simulink model "Manager_1"  (R2025b)
settings: configuration reference "code" (kept outside this file)
undefined symbols (not defined in the file or in its folder): Button, buttonValue, TsControl
settings Model: DataDictionary=test.sldd  Creator=rpumpo  LastModifiedBy=rpumpo
settings ConfigSetRef: SourceName=code

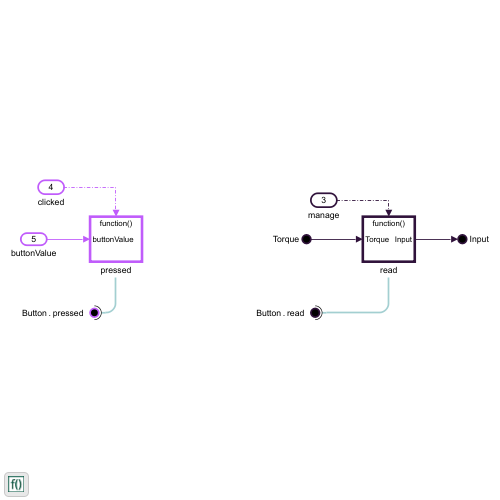
[thumbnail: Simulink's stored preview of the top-level diagram]
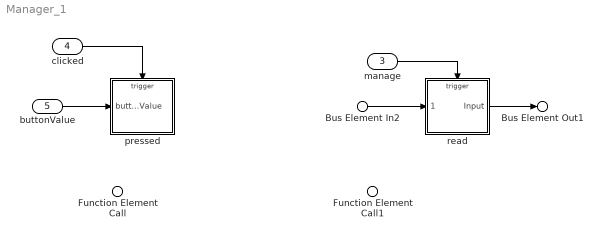
== system Manager_1 ==
  Function Element Call1 : Inport  AllowServiceAccess=on  PortName=Button  Element=read
  Function Element Call : Inport  AllowServiceAccess=on  PortName=Button  Element=pressed
  Bus Element In2 : Inport  Port=2  PortName=Torque
  manage : Inport  Port=3  SampleTime=TsControl  OutputFunctionCall=on
  clicked : Inport  Port=4  OutputFunctionCall=on
  buttonValue : Inport  Port=5
  pressed : Subsystem
  read : Subsystem
  Bus Element Out1 : Outport  PortName=Input
  wires:
  manage/1 -> read/Trigger
  read/1(Input) -> Bus Element Out1/1
  Bus Element In2/1 -> read/1(Torque)
  clicked/1 -> pressed/Trigger
  buttonValue/1 -> pressed/1(buttonValue)

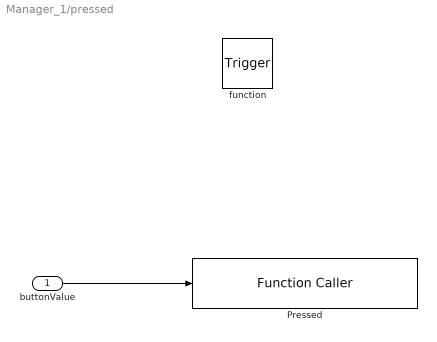
== system Manager_1/pressed ==
  buttonValue : Inport
  function : TriggerPort  TriggerType=function-call  VariantControl=(inherit)
  Pressed : FunctionCaller  FunctionPrototype=Button.pressed(buttonValue)  InputArgumentSpecifications=<Enter example>  OutputArgumentSpecifications=<Enter example>
  wires:
  buttonValue/1 -> Pressed/1

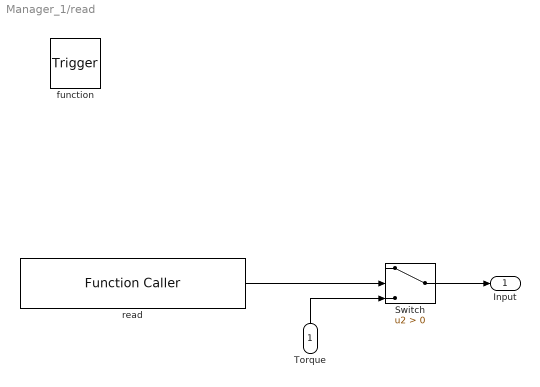
== system Manager_1/read ==
  Torque : Inport
  function : TriggerPort  TriggerType=function-call  VariantControl=(inherit)
  Switch : Switch  Criteria=u2 > Threshold  SaturateOnIntegerOverflow=off  InputSameDT=off
  read : FunctionCaller  FunctionPrototype=buttonPressed = Button.read()  InputArgumentSpecifications=<Enter example>  OutputArgumentSpecifications=<Enter example>
  Input : Outport
  wires:
  read/1 -> Switch/2
  Switch/1 -> Input/1
  Torque/1 -> Switch/3
